simulink model "ThdRwLtStBkReclnTrgtPosSelc"  (R2018b)
settings: Solver=FixedStepDiscrete  StartTime=0.0  StopTime=10.0  RelTol=1e-3
undefined symbols (not defined in the file or in its folder): KeSMSw6sAcsEntryThdRwLtStBkReclnUpwdDnwdPos_Val, KeSMSw6sAcsEntryThdRwLtStBkReclnUpwdDnwdPosMax_Val, KeSMSw6sAcsEntryThdRwLtStBkReclnUpwdDnwdPosMin_Val, KeSMSw6sLugThdRwLtStBkReclnUpwdDnwdPos_Val, KeSMSw6sLugThdRwLtStBkReclnUpwdDnwdPosMax_Val, KeSMSw6sLugThdRwLtStBkReclnUpwdDnwdPosMin_Val, KeSMSw6sVIPThdRwLtStBkReclnUpwdDnwdPos_Val, KeSMSw6sVIPThdRwLtStBkReclnUpwdDnwdPosMax_Val, KeSMSw6sVIPThdRwLtStBkReclnUpwdDnwdPosMin_Val, KeSMSwAcsEntryThdRwLtStBkReclnUpwdDnwdPos_Val, KeSMSwAcsEntryThdRwLtStBkReclnUpwdDnwdPosMax_Val, KeSMSwAcsEntryThdRwLtStBkReclnUpwdDnwdPosMin_Val, KeSMSwAcsMd32ThdRwLtBkReclnUpwdDnwdPos_Val, KeSMSwAcsMd32ThdRwLtBkReclnUpwdDnwdPosMax_Val, KeSMSwAcsMd32ThdRwLtBkReclnUpwdDnwdPosMin_Val, KeSMSwLugThdRwLtStBkReclnUpwdDnwdPos_Val, KeSMSwLugThdRwLtStBkReclnUpwdDnwdPosMax_Val, KeSMSwLugThdRwLtStBkReclnUpwdDnwdPosMin_Val, KeSMSwVIPThdRwLtStBkReclnUpwdDnwdPos_Val, KeSMSwVIPThdRwLtStBkReclnUpwdDnwdPosMax_Val, KeSMSwVIPThdRwLtStBkReclnUpwdDnwdPosMin_Val
libraries: TrgtPosSelcLib x5
settings Model: Creator=sn2xws  LastModifiedBy=sn2xws
settings Model: ModifiedHistory=|
  | 2024.6.25
  | V3.0.0 557模式流程V1.6
settings DataIOCC: SaveFormat=StructureWithTime
settings OptimizationCC: DefaultParameterBehavior=Inlined  EnhancedBackFolding=on  PassReuseOutputArgsAs=Individual arguments  ZeroExternalMemoryAtStartup=off  ZeroInternalMemoryAtStartup=off  OptimizeBlockOrder=speed  DifferentSizesBufferReuse=on  OptimizationCustomize=off
settings DebuggingCC: ParameterTunabilityLossMsg=error
settings SFSimCC: MATLABDynamicMemAlloc=off
settings RTWCC: SystemTargetFile=autosar.tlc  GenCodeOnly=on  TemplateMakefile=ert_default_tmf  Description=AUTOSAR  GenerateReport=on  IncludeHyperlinkInReport=on  LaunchReport=on  GenerateTraceInfo=on  GenerateTraceReport=on  GenerateTraceReportSl=on  GenerateTraceReportSf=on  GenerateTraceReportEml=on  GenerateCodeMetricsReport=on
settings CodeAppCC: ForceParamTrailComments=on  IgnoreCustomStorageClasses=off  OperatorAnnotations=on  SimulinkDataObjDesc=on  SFDataObjDesc=on  InsertBlockDesc=on
settings STFCustomTargetCC: TargetLangStandard=C99 (ISO)  MultiwordLength=256  ParMdlRefBuildCompliant=on  CompOptLevelCompliant=on  IncludeMdlTerminateFcn=off  CombineOutputUpdateFcns=on  SuppressErrorStatus=on  ERTCustomFileBanners=on  SupportNonFinite=off  SupportComplex=off  SupportContinuousTime=off  SupportNonInlinedSFcns=off  RemoveResetFunc=on  MATLABClassNameForMDSCustomization=Simulink.SoftwareTarget.ERTCustomization  AutosarCompliant=on  UseToolchainInfoCompliant=on  LookupTableObjectStructAxisOrder=2,1,3,4,...  LUTObjectStructOrderEvenSpacing=Size,Table,Breakpoints  SystemTargetFile=autosar.tlc
settings ERTTargetCC: TargetLangStandard=C99 (ISO)  ConcurrentExecutionCompliant=off  IncludeMdlTerminateFcn=off  SuppressErrorStatus=on  SupportNonFinite=off  SupportComplex=off  ModelStepFunctionPrototypeControlCompliant=off  CPPClassGenCompliant=off  AutosarCompliant=on  LookupTableObjectStructAxisOrder=2,1,3,4,...  LUTObjectStructOrderEvenSpacing=Size,Table,Breakpoints  InlinedParameterPlacement=NonHierarchical  ERTCustomFileTemplate=example_file_process.tlc  ERTFilePackagingFormat=Compact

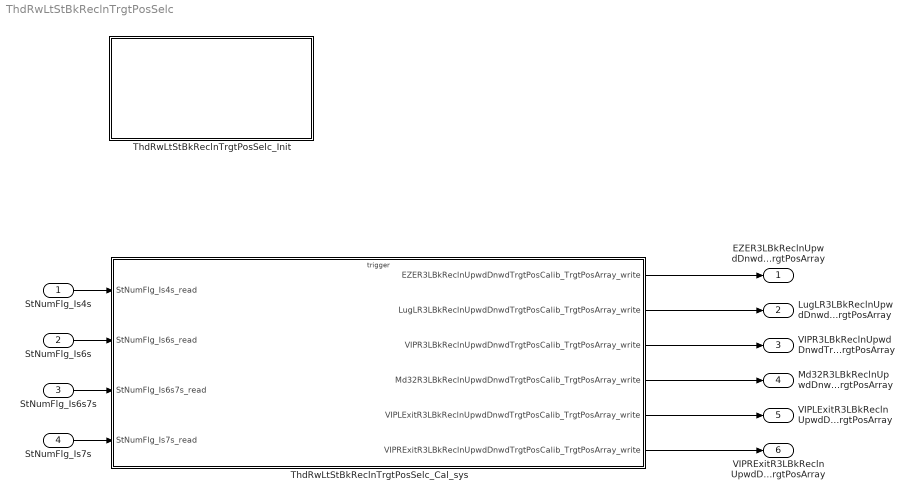
== system ThdRwLtStBkReclnTrgtPosSelc ==
  StNumFlg_Is4s : Inport  OutDataTypeStr=boolean  PortDimensions=1
  StNumFlg_Is6s : Inport  Port=2  OutDataTypeStr=boolean  PortDimensions=1
  StNumFlg_Is6s7s : Inport  Port=3  OutDataTypeStr=boolean  PortDimensions=1
  StNumFlg_Is7s : Inport  Port=4  OutDataTypeStr=boolean  PortDimensions=1
  ThdRwLtStBkReclnTrgtPosSelc_Cal_sys : Subsystem
  ThdRwLtStBkReclnTrgtPosSelc_Init : Subsystem
  EZER3LBkReclnUpwdDnwdTrgtPosCalib_TrgtPosArray : Outport  Description=|  OutDataTypeStr=uint16  PortDimensions=3
      | 0:Pos
      | 1:Max
      | 2:Min
  LugLR3LBkReclnUpwdDnwdTrgtPosCalib_TrgtPosArray : Outport  Description=|  Port=2  OutDataTypeStr=uint16  PortDimensions=3
      | 0:Pos
      | 1:Max
      | 2:Min
  VIPR3LBkReclnUpwdDnwdTrgtPosCalib_TrgtPosArray : Outport  Description=|  Port=3  OutDataTypeStr=uint16  PortDimensions=3
      | 0:Pos
      | 1:Max
      | 2:Min
  Md32R3LBkReclnUpwdDnwdTrgtPosCalib_TrgtPosArray : Outport  Description=|  Port=4  OutDataTypeStr=uint16  PortDimensions=3
      | 0:Pos
      | 1:Max
      | 2:Min
  VIPLExitR3LBkReclnUpwdDnwdTrgtPosCalib_TrgtPosArray : Outport  Description=|  Port=5  OutDataTypeStr=uint16  PortDimensions=3
      | 0:Pos
      | 1:Max
      | 2:Min
  VIPRExitR3LBkReclnUpwdDnwdTrgtPosCalib_TrgtPosArray : Outport  Description=|  Port=6  OutDataTypeStr=uint16  PortDimensions=3
      | 0:Pos
      | 1:Max
      | 2:Min
  wires:
  StNumFlg_Is4s/1 -> ThdRwLtStBkReclnTrgtPosSelc_Cal_sys/1(StNumFlg_Is4s_read)
  StNumFlg_Is6s/1 -> ThdRwLtStBkReclnTrgtPosSelc_Cal_sys/2(StNumFlg_Is6s_read)
  StNumFlg_Is6s7s/1 -> ThdRwLtStBkReclnTrgtPosSelc_Cal_sys/3(StNumFlg_Is6s7s_read)
  StNumFlg_Is7s/1 -> ThdRwLtStBkReclnTrgtPosSelc_Cal_sys/4(StNumFlg_Is7s_read)
  ThdRwLtStBkReclnTrgtPosSelc_Cal_sys/1(EZER3LBkReclnUpwdDnwdTrgtPosCalib_TrgtPosArray_write) -> EZER3LBkReclnUpwdDnwdTrgtPosCalib_TrgtPosArray/1
  ThdRwLtStBkReclnTrgtPosSelc_Cal_sys/2(LugLR3LBkReclnUpwdDnwdTrgtPosCalib_TrgtPosArray_write) -> LugLR3LBkReclnUpwdDnwdTrgtPosCalib_TrgtPosArray/1
  ThdRwLtStBkReclnTrgtPosSelc_Cal_sys/3(VIPR3LBkReclnUpwdDnwdTrgtPosCalib_TrgtPosArray_write) -> VIPR3LBkReclnUpwdDnwdTrgtPosCalib_TrgtPosArray/1
  ThdRwLtStBkReclnTrgtPosSelc_Cal_sys/4(Md32R3LBkReclnUpwdDnwdTrgtPosCalib_TrgtPosArray_write) -> Md32R3LBkReclnUpwdDnwdTrgtPosCalib_TrgtPosArray/1
  ThdRwLtStBkReclnTrgtPosSelc_Cal_sys/5(VIPLExitR3LBkReclnUpwdDnwdTrgtPosCalib_TrgtPosArray_write) -> VIPLExitR3LBkReclnUpwdDnwdTrgtPosCalib_TrgtPosArray/1
  ThdRwLtStBkReclnTrgtPosSelc_Cal_sys/6(VIPRExitR3LBkReclnUpwdDnwdTrgtPosCalib_TrgtPosArray_write) -> VIPRExitR3LBkReclnUpwdDnwdTrgtPosCalib_TrgtPosArray/1

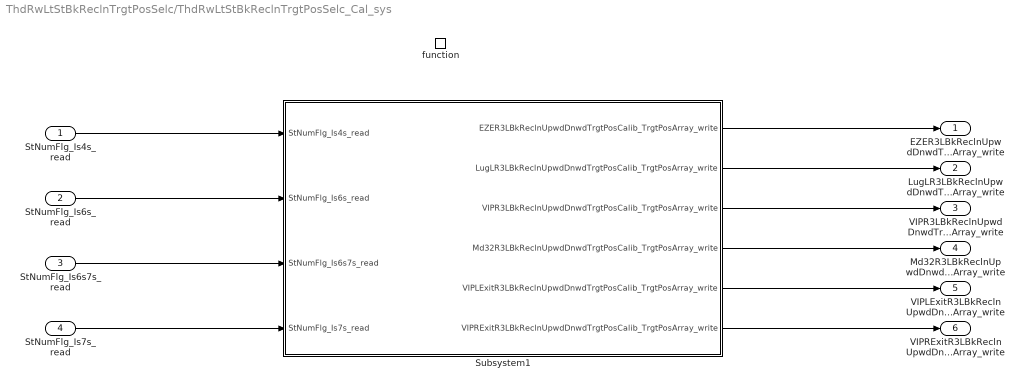
== system ThdRwLtStBkReclnTrgtPosSelc/ThdRwLtStBkReclnTrgtPosSelc_Cal_sys ==
  StNumFlg_Is4s_read : Inport
  StNumFlg_Is6s_read : Inport  Port=2
  StNumFlg_Is6s7s_read : Inport  Port=3
  StNumFlg_Is7s_read : Inport  Port=4
  function : TriggerPort  TriggerType=function-call  IsSimulinkFunction=on  FunctionName=ThdRwLtStBkReclnTrgtPosSelc_Cal  VariantControl=(inherit)
  Subsystem1 : Subsystem
  EZER3LBkReclnUpwdDnwdTrgtPosCalib_TrgtPosArray_write : Outport
      settings: EnsureOutportIsVirtual=on
  LugLR3LBkReclnUpwdDnwdTrgtPosCalib_TrgtPosArray_write : Outport  Port=2
      settings: EnsureOutportIsVirtual=on
  VIPR3LBkReclnUpwdDnwdTrgtPosCalib_TrgtPosArray_write : Outport  Port=3
      settings: EnsureOutportIsVirtual=on
  Md32R3LBkReclnUpwdDnwdTrgtPosCalib_TrgtPosArray_write : Outport  Port=4
      settings: EnsureOutportIsVirtual=on
  VIPLExitR3LBkReclnUpwdDnwdTrgtPosCalib_TrgtPosArray_write : Outport  Port=5
      settings: EnsureOutportIsVirtual=on
  VIPRExitR3LBkReclnUpwdDnwdTrgtPosCalib_TrgtPosArray_write : Outport  Port=6
      settings: EnsureOutportIsVirtual=on
  wires:
  Subsystem1/1(EZER3LBkReclnUpwdDnwdTrgtPosCalib_TrgtPosArray_write) -> EZER3LBkReclnUpwdDnwdTrgtPosCalib_TrgtPosArray_write/1
  Subsystem1/2(LugLR3LBkReclnUpwdDnwdTrgtPosCalib_TrgtPosArray_write) -> LugLR3LBkReclnUpwdDnwdTrgtPosCalib_TrgtPosArray_write/1
  Subsystem1/3(VIPR3LBkReclnUpwdDnwdTrgtPosCalib_TrgtPosArray_write) -> VIPR3LBkReclnUpwdDnwdTrgtPosCalib_TrgtPosArray_write/1
  StNumFlg_Is4s_read/1 -> Subsystem1/1(StNumFlg_Is4s_read)
  StNumFlg_Is6s_read/1 -> Subsystem1/2(StNumFlg_Is6s_read)
  StNumFlg_Is6s7s_read/1 -> Subsystem1/3(StNumFlg_Is6s7s_read)
  StNumFlg_Is7s_read/1 -> Subsystem1/4(StNumFlg_Is7s_read)
  Subsystem1/4(Md32R3LBkReclnUpwdDnwdTrgtPosCalib_TrgtPosArray_write) -> Md32R3LBkReclnUpwdDnwdTrgtPosCalib_TrgtPosArray_write/1
  Subsystem1/5(VIPLExitR3LBkReclnUpwdDnwdTrgtPosCalib_TrgtPosArray_write) -> VIPLExitR3LBkReclnUpwdDnwdTrgtPosCalib_TrgtPosArray_write/1
  Subsystem1/6(VIPRExitR3LBkReclnUpwdDnwdTrgtPosCalib_TrgtPosArray_write) -> VIPRExitR3LBkReclnUpwdDnwdTrgtPosCalib_TrgtPosArray_write/1

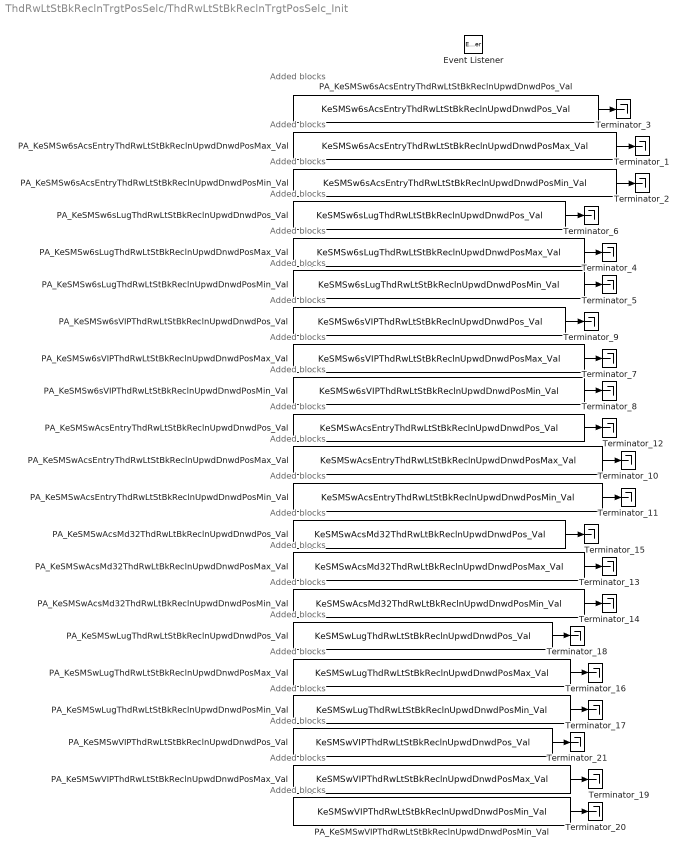
== system ThdRwLtStBkReclnTrgtPosSelc/ThdRwLtStBkReclnTrgtPosSelc_Init ==
  note: Added blocks
  note: Added blocks
  note: Added blocks
  note: Added blocks
  note: Added blocks
  note: Added blocks
  note: Added blocks
  note: Added blocks
  note: Added blocks
  note: Added blocks
  note: Added blocks
  note: Added blocks
  note: Added blocks
  note: Added blocks
  note: Added blocks
  note: Added blocks
  note: Added blocks
  note: Added blocks
  note: Added blocks
  note: Added blocks
  note: Added blocks
  Event Listener : EventListener  EventName=reset
  PA_KeSMSw6sAcsEntryThdRwLtStBkReclnUpwdDnwdPosMax_Val : Constant  Value=KeSMSw6sAcsEntryThdRwLtStBkReclnUpwdDnwdPosMax_Val
  PA_KeSMSw6sAcsEntryThdRwLtStBkReclnUpwdDnwdPosMin_Val : Constant  Value=KeSMSw6sAcsEntryThdRwLtStBkReclnUpwdDnwdPosMin_Val
  PA_KeSMSw6sAcsEntryThdRwLtStBkReclnUpwdDnwdPos_Val : Constant  Value=KeSMSw6sAcsEntryThdRwLtStBkReclnUpwdDnwdPos_Val
  PA_KeSMSw6sLugThdRwLtStBkReclnUpwdDnwdPosMax_Val : Constant  Value=KeSMSw6sLugThdRwLtStBkReclnUpwdDnwdPosMax_Val
  PA_KeSMSw6sLugThdRwLtStBkReclnUpwdDnwdPosMin_Val : Constant  Value=KeSMSw6sLugThdRwLtStBkReclnUpwdDnwdPosMin_Val
  PA_KeSMSw6sLugThdRwLtStBkReclnUpwdDnwdPos_Val : Constant  Value=KeSMSw6sLugThdRwLtStBkReclnUpwdDnwdPos_Val
  PA_KeSMSw6sVIPThdRwLtStBkReclnUpwdDnwdPosMax_Val : Constant  Value=KeSMSw6sVIPThdRwLtStBkReclnUpwdDnwdPosMax_Val
  PA_KeSMSw6sVIPThdRwLtStBkReclnUpwdDnwdPosMin_Val : Constant  Value=KeSMSw6sVIPThdRwLtStBkReclnUpwdDnwdPosMin_Val
  PA_KeSMSw6sVIPThdRwLtStBkReclnUpwdDnwdPos_Val : Constant  Value=KeSMSw6sVIPThdRwLtStBkReclnUpwdDnwdPos_Val
  PA_KeSMSwAcsEntryThdRwLtStBkReclnUpwdDnwdPosMax_Val : Constant  Value=KeSMSwAcsEntryThdRwLtStBkReclnUpwdDnwdPosMax_Val
  PA_KeSMSwAcsEntryThdRwLtStBkReclnUpwdDnwdPosMin_Val : Constant  Value=KeSMSwAcsEntryThdRwLtStBkReclnUpwdDnwdPosMin_Val
  PA_KeSMSwAcsEntryThdRwLtStBkReclnUpwdDnwdPos_Val : Constant  Value=KeSMSwAcsEntryThdRwLtStBkReclnUpwdDnwdPos_Val
  PA_KeSMSwAcsMd32ThdRwLtBkReclnUpwdDnwdPosMax_Val : Constant  Value=KeSMSwAcsMd32ThdRwLtBkReclnUpwdDnwdPosMax_Val
  PA_KeSMSwAcsMd32ThdRwLtBkReclnUpwdDnwdPosMin_Val : Constant  Value=KeSMSwAcsMd32ThdRwLtBkReclnUpwdDnwdPosMin_Val
  PA_KeSMSwAcsMd32ThdRwLtBkReclnUpwdDnwdPos_Val : Constant  Value=KeSMSwAcsMd32ThdRwLtBkReclnUpwdDnwdPos_Val
  PA_KeSMSwLugThdRwLtStBkReclnUpwdDnwdPosMax_Val : Constant  Value=KeSMSwLugThdRwLtStBkReclnUpwdDnwdPosMax_Val
  PA_KeSMSwLugThdRwLtStBkReclnUpwdDnwdPosMin_Val : Constant  Value=KeSMSwLugThdRwLtStBkReclnUpwdDnwdPosMin_Val
  PA_KeSMSwLugThdRwLtStBkReclnUpwdDnwdPos_Val : Constant  Value=KeSMSwLugThdRwLtStBkReclnUpwdDnwdPos_Val
  PA_KeSMSwVIPThdRwLtStBkReclnUpwdDnwdPosMax_Val : Constant  Value=KeSMSwVIPThdRwLtStBkReclnUpwdDnwdPosMax_Val
  PA_KeSMSwVIPThdRwLtStBkReclnUpwdDnwdPosMin_Val : Constant  Value=KeSMSwVIPThdRwLtStBkReclnUpwdDnwdPosMin_Val
  PA_KeSMSwVIPThdRwLtStBkReclnUpwdDnwdPos_Val : Constant  Value=KeSMSwVIPThdRwLtStBkReclnUpwdDnwdPos_Val
  Terminator_{1..21} (21 alike) : Terminator
  wires:
  PA_KeSMSw6sAcsEntryThdRwLtStBkReclnUpwdDnwdPosMax_Val/1 -> Terminator_1/1
  PA_KeSMSw6sAcsEntryThdRwLtStBkReclnUpwdDnwdPosMin_Val/1 -> Terminator_2/1
  PA_KeSMSw6sAcsEntryThdRwLtStBkReclnUpwdDnwdPos_Val/1 -> Terminator_3/1
  PA_KeSMSw6sLugThdRwLtStBkReclnUpwdDnwdPosMax_Val/1 -> Terminator_4/1
  PA_KeSMSw6sLugThdRwLtStBkReclnUpwdDnwdPosMin_Val/1 -> Terminator_5/1
  PA_KeSMSw6sLugThdRwLtStBkReclnUpwdDnwdPos_Val/1 -> Terminator_6/1
  PA_KeSMSw6sVIPThdRwLtStBkReclnUpwdDnwdPosMax_Val/1 -> Terminator_7/1
  PA_KeSMSw6sVIPThdRwLtStBkReclnUpwdDnwdPosMin_Val/1 -> Terminator_8/1
  PA_KeSMSw6sVIPThdRwLtStBkReclnUpwdDnwdPos_Val/1 -> Terminator_9/1
  PA_KeSMSwAcsEntryThdRwLtStBkReclnUpwdDnwdPosMax_Val/1 -> Terminator_10/1
  PA_KeSMSwAcsEntryThdRwLtStBkReclnUpwdDnwdPosMin_Val/1 -> Terminator_11/1
  PA_KeSMSwAcsEntryThdRwLtStBkReclnUpwdDnwdPos_Val/1 -> Terminator_12/1
  PA_KeSMSwAcsMd32ThdRwLtBkReclnUpwdDnwdPosMax_Val/1 -> Terminator_13/1
  PA_KeSMSwAcsMd32ThdRwLtBkReclnUpwdDnwdPosMin_Val/1 -> Terminator_14/1
  PA_KeSMSwAcsMd32ThdRwLtBkReclnUpwdDnwdPos_Val/1 -> Terminator_15/1
  PA_KeSMSwLugThdRwLtStBkReclnUpwdDnwdPosMax_Val/1 -> Terminator_16/1
  PA_KeSMSwLugThdRwLtStBkReclnUpwdDnwdPosMin_Val/1 -> Terminator_17/1
  PA_KeSMSwLugThdRwLtStBkReclnUpwdDnwdPos_Val/1 -> Terminator_18/1
  PA_KeSMSwVIPThdRwLtStBkReclnUpwdDnwdPosMax_Val/1 -> Terminator_19/1
  PA_KeSMSwVIPThdRwLtStBkReclnUpwdDnwdPosMin_Val/1 -> Terminator_20/1
  PA_KeSMSwVIPThdRwLtStBkReclnUpwdDnwdPos_Val/1 -> Terminator_21/1

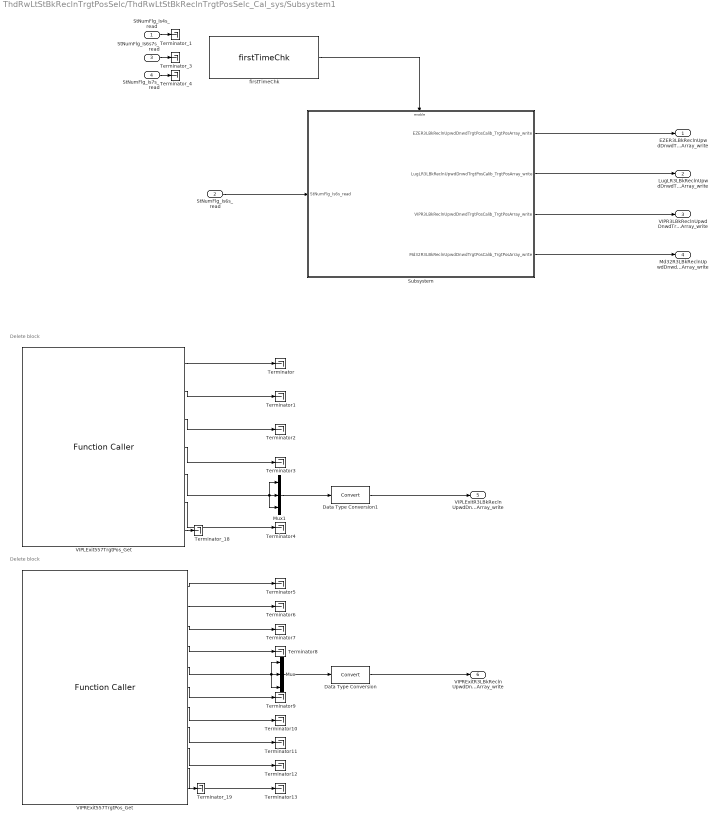
== system ThdRwLtStBkReclnTrgtPosSelc/ThdRwLtStBkReclnTrgtPosSelc_Cal_sys/Subsystem1 ==
  note: Delete block
  note: Delete block
  StNumFlg_Is4s_read : Inport
  StNumFlg_Is6s_read : Inport  Port=2
  StNumFlg_Is6s7s_read : Inport  Port=3
  StNumFlg_Is7s_read : Inport  Port=4
  Data Type Conversion : DataTypeConversion
  Data Type Conversion1 : DataTypeConversion
  Mux : Mux  Inputs=3
  Mux1 : Mux  Inputs=3
  Subsystem : Subsystem
  Terminator{,1..13} (14 alike) : Terminator
  Terminator_{1,3..4,18..19} (5 alike) : Terminator
  VIPLExit557TrgtPos_Get : FunctionCaller  FunctionPrototype=[SecRwLtStBkReclnTrgtPos,SecRwLtStZeroTrgtPos,SecRwLtStLgrstUpwdDnwdTrgtPos,SecRwLtStLgrstInwdOtwdTrgtPos,ThdRwLtStBkReclnTrgtPos,ThdRwLtStFwdBkwdTrgtPos,SecRwLtStFwdBkwdTrgtPos] = VIPLExit557TrgtPos_Get()  OutputArgumentSpecifications=uint16(1), uint16(1), uint16(1), uint16(1), uint16(1), uint16(1), uint16(1)
  VIPRExit557TrgtPos_Get : FunctionCaller  FunctionPrototype=[SecRwRtStBkReclnTrgtPos,SecRwRtStZeroTrgtPos,SecRwRtStLgrstUpwdDnwdTrgtPos,SecRwRtStLgrstInwdOtwdTrgtPos,ThdRwLtStBkReclnTrgtPos,ThdRwLtStFwdBkwdTrgtPos,ThdRwRtStBkReclnTrgtPos,ThdRwRtStFwdBkwdTrgtPos,PassStBkReclnTrgtPos,PassStFwdBkwdTrgtPos,SecRwRtStFwdBkwdTrgtPos] = VIPRExit557TrgtPos_Get()  OutputArgumentSpecifications=uint16(1), uint16(1), uint16(1), uint16(1), uint16(1), uint16(1), uint16(1), uint16(1), uint16(1), uint16(1), uint16(1)
  firstTimeChk : TrgtPosSelcLib/firstTimeChk  SystemSampleTime=-1
  EZER3LBkReclnUpwdDnwdTrgtPosCalib_TrgtPosArray_write : Outport
      settings: EnsureOutportIsVirtual=on
  LugLR3LBkReclnUpwdDnwdTrgtPosCalib_TrgtPosArray_write : Outport  Port=2
      settings: EnsureOutportIsVirtual=on
  VIPR3LBkReclnUpwdDnwdTrgtPosCalib_TrgtPosArray_write : Outport  Port=3
      settings: EnsureOutportIsVirtual=on
  Md32R3LBkReclnUpwdDnwdTrgtPosCalib_TrgtPosArray_write : Outport  Port=4
      settings: EnsureOutportIsVirtual=on
  VIPLExitR3LBkReclnUpwdDnwdTrgtPosCalib_TrgtPosArray_write : Outport  Port=5
      settings: EnsureOutportIsVirtual=on
  VIPRExitR3LBkReclnUpwdDnwdTrgtPosCalib_TrgtPosArray_write : Outport  Port=6
      settings: EnsureOutportIsVirtual=on
  wires:
  StNumFlg_Is6s7s_read/1 -> Terminator_3/1
  StNumFlg_Is4s_read/1 -> Terminator_1/1
  StNumFlg_Is6s_read/1 -> Subsystem/1(StNumFlg_Is6s_read)
  Subsystem/2(LugLR3LBkReclnUpwdDnwdTrgtPosCalib_TrgtPosArray_write) -> LugLR3LBkReclnUpwdDnwdTrgtPosCalib_TrgtPosArray_write/1
  firstTimeChk/1 -> Subsystem/Enable
  StNumFlg_Is7s_read/1 -> Terminator_4/1
  Subsystem/3(VIPR3LBkReclnUpwdDnwdTrgtPosCalib_TrgtPosArray_write) -> VIPR3LBkReclnUpwdDnwdTrgtPosCalib_TrgtPosArray_write/1
  Subsystem/1(EZER3LBkReclnUpwdDnwdTrgtPosCalib_TrgtPosArray_write) -> EZER3LBkReclnUpwdDnwdTrgtPosCalib_TrgtPosArray_write/1
  Subsystem/4(Md32R3LBkReclnUpwdDnwdTrgtPosCalib_TrgtPosArray_write) -> Md32R3LBkReclnUpwdDnwdTrgtPosCalib_TrgtPosArray_write/1
  VIPRExit557TrgtPos_Get/5 -> Mux/1, Mux/3, Mux/2
  Mux/1 -> Data Type Conversion/1
  Data Type Conversion/1 -> VIPRExitR3LBkReclnUpwdDnwdTrgtPosCalib_TrgtPosArray_write/1
  Data Type Conversion1/1 -> VIPLExitR3LBkReclnUpwdDnwdTrgtPosCalib_TrgtPosArray_write/1
  Mux1/1 -> Data Type Conversion1/1
  VIPLExit557TrgtPos_Get/5 -> Mux1/1, Mux1/2, Mux1/3
  VIPLExit557TrgtPos_Get/1 -> Terminator/1
  VIPLExit557TrgtPos_Get/2 -> Terminator1/1
  VIPLExit557TrgtPos_Get/3 -> Terminator2/1
  VIPLExit557TrgtPos_Get/4 -> Terminator3/1
  VIPLExit557TrgtPos_Get/6 -> Terminator4/1
  VIPRExit557TrgtPos_Get/1 -> Terminator5/1
  VIPRExit557TrgtPos_Get/2 -> Terminator6/1
  VIPRExit557TrgtPos_Get/3 -> Terminator7/1
  VIPRExit557TrgtPos_Get/4 -> Terminator8/1
  VIPRExit557TrgtPos_Get/6 -> Terminator9/1
  VIPRExit557TrgtPos_Get/7 -> Terminator10/1
  VIPRExit557TrgtPos_Get/8 -> Terminator11/1
  VIPRExit557TrgtPos_Get/9 -> Terminator12/1
  VIPRExit557TrgtPos_Get/10 -> Terminator13/1
  VIPLExit557TrgtPos_Get/7 -> Terminator_18/1
  VIPRExit557TrgtPos_Get/11 -> Terminator_19/1

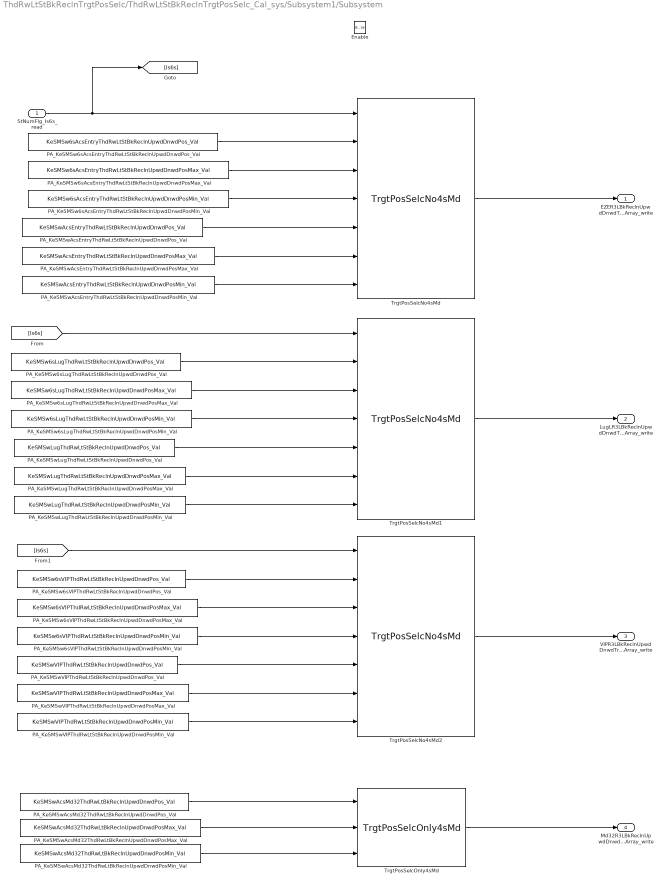
== system ThdRwLtStBkReclnTrgtPosSelc/ThdRwLtStBkReclnTrgtPosSelc_Cal_sys/Subsystem1/Subsystem ==
  StNumFlg_Is6s_read : Inport
  Enable : EnablePort
  PA_KeSMSw6sAcsEntryThdRwLtStBkReclnUpwdDnwdPosMax_Val : Constant  Value=KeSMSw6sAcsEntryThdRwLtStBkReclnUpwdDnwdPosMax_Val
  PA_KeSMSw6sAcsEntryThdRwLtStBkReclnUpwdDnwdPosMin_Val : Constant  Value=KeSMSw6sAcsEntryThdRwLtStBkReclnUpwdDnwdPosMin_Val
  PA_KeSMSw6sAcsEntryThdRwLtStBkReclnUpwdDnwdPos_Val : Constant  Value=KeSMSw6sAcsEntryThdRwLtStBkReclnUpwdDnwdPos_Val
  PA_KeSMSw6sLugThdRwLtStBkReclnUpwdDnwdPosMax_Val : Constant  Value=KeSMSw6sLugThdRwLtStBkReclnUpwdDnwdPosMax_Val
  PA_KeSMSw6sLugThdRwLtStBkReclnUpwdDnwdPosMin_Val : Constant  Value=KeSMSw6sLugThdRwLtStBkReclnUpwdDnwdPosMin_Val
  PA_KeSMSw6sLugThdRwLtStBkReclnUpwdDnwdPos_Val : Constant  Value=KeSMSw6sLugThdRwLtStBkReclnUpwdDnwdPos_Val
  PA_KeSMSw6sVIPThdRwLtStBkReclnUpwdDnwdPosMax_Val : Constant  Value=KeSMSw6sVIPThdRwLtStBkReclnUpwdDnwdPosMax_Val
  PA_KeSMSw6sVIPThdRwLtStBkReclnUpwdDnwdPosMin_Val : Constant  Value=KeSMSw6sVIPThdRwLtStBkReclnUpwdDnwdPosMin_Val
  PA_KeSMSw6sVIPThdRwLtStBkReclnUpwdDnwdPos_Val : Constant  Value=KeSMSw6sVIPThdRwLtStBkReclnUpwdDnwdPos_Val
  PA_KeSMSwAcsEntryThdRwLtStBkReclnUpwdDnwdPosMax_Val : Constant  Value=KeSMSwAcsEntryThdRwLtStBkReclnUpwdDnwdPosMax_Val
  PA_KeSMSwAcsEntryThdRwLtStBkReclnUpwdDnwdPosMin_Val : Constant  Value=KeSMSwAcsEntryThdRwLtStBkReclnUpwdDnwdPosMin_Val
  PA_KeSMSwAcsEntryThdRwLtStBkReclnUpwdDnwdPos_Val : Constant  Value=KeSMSwAcsEntryThdRwLtStBkReclnUpwdDnwdPos_Val
  PA_KeSMSwAcsMd32ThdRwLtBkReclnUpwdDnwdPosMax_Val : Constant  Value=KeSMSwAcsMd32ThdRwLtBkReclnUpwdDnwdPosMax_Val
  PA_KeSMSwAcsMd32ThdRwLtBkReclnUpwdDnwdPosMin_Val : Constant  Value=KeSMSwAcsMd32ThdRwLtBkReclnUpwdDnwdPosMin_Val
  PA_KeSMSwAcsMd32ThdRwLtBkReclnUpwdDnwdPos_Val : Constant  Value=KeSMSwAcsMd32ThdRwLtBkReclnUpwdDnwdPos_Val
  PA_KeSMSwLugThdRwLtStBkReclnUpwdDnwdPosMax_Val : Constant  Value=KeSMSwLugThdRwLtStBkReclnUpwdDnwdPosMax_Val
  PA_KeSMSwLugThdRwLtStBkReclnUpwdDnwdPosMin_Val : Constant  Value=KeSMSwLugThdRwLtStBkReclnUpwdDnwdPosMin_Val
  PA_KeSMSwLugThdRwLtStBkReclnUpwdDnwdPos_Val : Constant  Value=KeSMSwLugThdRwLtStBkReclnUpwdDnwdPos_Val
  PA_KeSMSwVIPThdRwLtStBkReclnUpwdDnwdPosMax_Val : Constant  Value=KeSMSwVIPThdRwLtStBkReclnUpwdDnwdPosMax_Val
  PA_KeSMSwVIPThdRwLtStBkReclnUpwdDnwdPosMin_Val : Constant  Value=KeSMSwVIPThdRwLtStBkReclnUpwdDnwdPosMin_Val
  PA_KeSMSwVIPThdRwLtStBkReclnUpwdDnwdPos_Val : Constant  Value=KeSMSwVIPThdRwLtStBkReclnUpwdDnwdPos_Val
  TrgtPosSelcNo4sMd : TrgtPosSelcLib/TrgtPosSelcNo4sMd  SystemSampleTime=-1
  TrgtPosSelcNo4sMd1 : TrgtPosSelcLib/TrgtPosSelcNo4sMd  SystemSampleTime=-1
  TrgtPosSelcNo4sMd2 : TrgtPosSelcLib/TrgtPosSelcNo4sMd  SystemSampleTime=-1
  TrgtPosSelcOnly4sMd : TrgtPosSelcLib/TrgtPosSelcOnly4sMd  SystemSampleTime=-1
  EZER3LBkReclnUpwdDnwdTrgtPosCalib_TrgtPosArray_write : Outport
      settings: EnsureOutportIsVirtual=on
  LugLR3LBkReclnUpwdDnwdTrgtPosCalib_TrgtPosArray_write : Outport  Port=2
      settings: EnsureOutportIsVirtual=on
  VIPR3LBkReclnUpwdDnwdTrgtPosCalib_TrgtPosArray_write : Outport  Port=3
      settings: EnsureOutportIsVirtual=on
  Md32R3LBkReclnUpwdDnwdTrgtPosCalib_TrgtPosArray_write : Outport  Port=4
      settings: EnsureOutportIsVirtual=on
  wires:
  StNumFlg_Is6s_read/1 -> [Is6s], TrgtPosSelcNo4sMd/1
  TrgtPosSelcNo4sMd1/1 -> LugLR3LBkReclnUpwdDnwdTrgtPosCalib_TrgtPosArray_write/1
  TrgtPosSelcNo4sMd2/1 -> VIPR3LBkReclnUpwdDnwdTrgtPosCalib_TrgtPosArray_write/1
  TrgtPosSelcNo4sMd/1 -> EZER3LBkReclnUpwdDnwdTrgtPosCalib_TrgtPosArray_write/1
  [Is6s] -> TrgtPosSelcNo4sMd1/1
  PA_KeSMSw6sAcsEntryThdRwLtStBkReclnUpwdDnwdPosMax_Val/1 -> TrgtPosSelcNo4sMd/3
  PA_KeSMSw6sAcsEntryThdRwLtStBkReclnUpwdDnwdPosMin_Val/1 -> TrgtPosSelcNo4sMd/4
  PA_KeSMSw6sAcsEntryThdRwLtStBkReclnUpwdDnwdPos_Val/1 -> TrgtPosSelcNo4sMd/2
  PA_KeSMSw6sLugThdRwLtStBkReclnUpwdDnwdPosMax_Val/1 -> TrgtPosSelcNo4sMd1/3
  PA_KeSMSw6sLugThdRwLtStBkReclnUpwdDnwdPos_Val/1 -> TrgtPosSelcNo4sMd1/2
  PA_KeSMSw6sLugThdRwLtStBkReclnUpwdDnwdPosMin_Val/1 -> TrgtPosSelcNo4sMd1/4
  [Is6s] -> TrgtPosSelcNo4sMd2/1
  PA_KeSMSw6sVIPThdRwLtStBkReclnUpwdDnwdPosMax_Val/1 -> TrgtPosSelcNo4sMd2/3
  PA_KeSMSw6sVIPThdRwLtStBkReclnUpwdDnwdPos_Val/1 -> TrgtPosSelcNo4sMd2/2
  PA_KeSMSw6sVIPThdRwLtStBkReclnUpwdDnwdPosMin_Val/1 -> TrgtPosSelcNo4sMd2/4
  PA_KeSMSwAcsEntryThdRwLtStBkReclnUpwdDnwdPosMax_Val/1 -> TrgtPosSelcNo4sMd/6
  PA_KeSMSwAcsEntryThdRwLtStBkReclnUpwdDnwdPosMin_Val/1 -> TrgtPosSelcNo4sMd/7
  PA_KeSMSwAcsEntryThdRwLtStBkReclnUpwdDnwdPos_Val/1 -> TrgtPosSelcNo4sMd/5
  PA_KeSMSwLugThdRwLtStBkReclnUpwdDnwdPosMax_Val/1 -> TrgtPosSelcNo4sMd1/6
  PA_KeSMSwLugThdRwLtStBkReclnUpwdDnwdPosMin_Val/1 -> TrgtPosSelcNo4sMd1/7
  PA_KeSMSwLugThdRwLtStBkReclnUpwdDnwdPos_Val/1 -> TrgtPosSelcNo4sMd1/5
  PA_KeSMSwVIPThdRwLtStBkReclnUpwdDnwdPosMax_Val/1 -> TrgtPosSelcNo4sMd2/6
  PA_KeSMSwVIPThdRwLtStBkReclnUpwdDnwdPos_Val/1 -> TrgtPosSelcNo4sMd2/5
  PA_KeSMSwVIPThdRwLtStBkReclnUpwdDnwdPosMin_Val/1 -> TrgtPosSelcNo4sMd2/7
  PA_KeSMSwAcsMd32ThdRwLtBkReclnUpwdDnwdPosMin_Val/1 -> TrgtPosSelcOnly4sMd/3
  PA_KeSMSwAcsMd32ThdRwLtBkReclnUpwdDnwdPosMax_Val/1 -> TrgtPosSelcOnly4sMd/2
  PA_KeSMSwAcsMd32ThdRwLtBkReclnUpwdDnwdPos_Val/1 -> TrgtPosSelcOnly4sMd/1
  TrgtPosSelcOnly4sMd/1 -> Md32R3LBkReclnUpwdDnwdTrgtPosCalib_TrgtPosArray_write/1
